simulink model "simulate_DSBLC_SDRreceiver"  (R2017a)
settings: Solver=VariableStepAuto  StartTime=0.0  StopTime=.01  RelTol=1e-3
InitFcn:
  | fs = 1e5;
  | frameSize = 1000;
libraries: dspsrcs4 x2, commchan3 x1
settings Model: Creator=prust  LastModifiedBy=prust

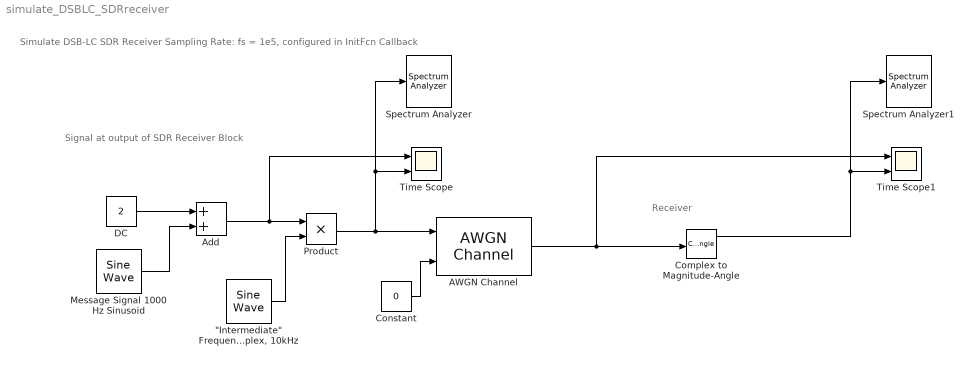
== system simulate_DSBLC_SDRreceiver ==
  note: Receiver
  note: Simulate DSB-LC SDR Receiver
      | Sampling Rate: fs = 1e5, configured in InitFcn Callback
  note: Signal at output of SDR Receiver Block
  "\"Intermediate\" Frequency Complex, 10kHz" : dspsrcs4/Sine Wave  Amplitude=1  Frequency=10e3  Phase=0  SampleMode=Discrete  OutComplex=Complex  CompMethod=Trigonometric fcn  TableSize=Speed  SampleTime=1/fs  SamplesPerFrame=frameSize  ResetState=Restart at time zero  OutputFrames=off  dataType=double  wordLen=16  udDataType=sfix(16)  fracBitsMode=Best precision  numFracBits=15  OutDataTypeStr=double  LastOutDataTypeStr=double
  AWGN Channel : commchan3/AWGN Channel  InputProcessing=Columns as channels (frame based)  seed=67  noiseMode=Variance from port  EbNodB=10  EsNodB=10  SNRdB=10  bitsPerSym=1  Ps=1  Tsym=1  variance=1
  Add : Sum
  Complex to Magnitude-Angle : ComplexToMagnitudeAngle
  Constant : Constant  Value=0
  DC : Constant  Value=2
  Message Signal 1000 Hz Sinusoid : dspsrcs4/Sine Wave  Amplitude=1  Frequency=1000  Phase=0  SampleMode=Discrete  OutComplex=Real  CompMethod=Trigonometric fcn  TableSize=Speed  SampleTime=1/fs  SamplesPerFrame=frameSize  ResetState=Restart at time zero  OutputFrames=off  dataType=double  wordLen=16  udDataType=sfix(16)  fracBitsMode=Best precision  numFracBits=15  OutDataTypeStr=double  LastOutDataTypeStr=double
  Product : Product
  Spectrum Analyzer : SpectrumAnalyzer
  Spectrum Analyzer1 : SpectrumAnalyzer
  Time Scope : Scope  NumInputPorts=2
  Time Scope1 : Scope  NumInputPorts=2
  wires:
  "\"Intermediate\" Frequency Complex, 10kHz"/1 -> Product/2
  Constant/1 -> AWGN Channel/2
  Product/1 -> AWGN Channel/1, Spectrum Analyzer/1, Time Scope/2
  AWGN Channel/1 -> Time Scope1/1, Complex to Magnitude-Angle/1
  Message Signal 1000 Hz Sinusoid/1 -> Add/2
  Add/1 -> Time Scope/1, Product/1
  DC/1 -> Add/1
  Complex to Magnitude-Angle/1 -> Time Scope1/2, Spectrum Analyzer1/1
